simulink model "TRIMRcam"  (R2025b)
settings: Solver=VariableStepAuto  StartTime=0.0  StopTime=10.0  RelTol=1e-3
values from neighbouring files (symbols this model uses):
  UStar = ZStar(10:16)    [trim.m]
settings Model: Creator=smthejaswini  LastModifiedBy=smthejaswini

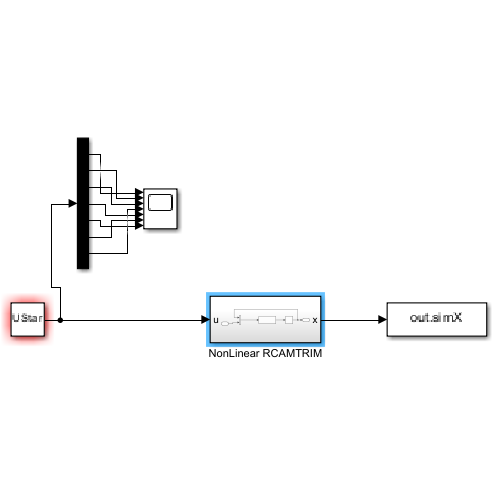
[thumbnail: Simulink's stored preview of the top-level diagram]
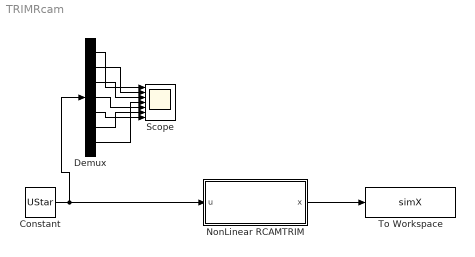
== system TRIMRcam ==
  Constant : Constant  Value=UStar
  Demux : Demux  Outputs=7
  NonLinear RCAMTRIM : Subsystem
  Scope : Scope  NumInputPorts=7
  To Workspace : ToWorkspace  VariableName=simX  SaveFormat=Timeseries  SampleTime=-1
  wires:
  Constant/1 -> NonLinear RCAMTRIM/1(u), Demux/1
  Demux/1 -> Scope/1
  Demux/2 -> Scope/2
  Demux/3 -> Scope/3
  Demux/4 -> Scope/5
  Demux/5 -> Scope/7
  Demux/6 -> Scope/6
  Demux/7 -> Scope/4
  NonLinear RCAMTRIM/1(x) -> To Workspace/1

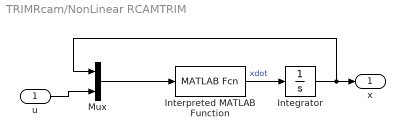
== system TRIMRcam/NonLinear RCAMTRIM ==
  u : Inport
  Integrator : Integrator
  Interpreted MATLAB Function : MATLABFcn
  Mux : Mux  Inputs=2
  x : Outport
  wires:
  u/1 -> Mux/2
  Mux/1 -> Interpreted MATLAB Function/1
  Interpreted MATLAB Function/1 -> Integrator/1  "xdot"
  Integrator/1 -> Mux/1, x/1
